simulink model "Fuzzy_System"  (R2024b)
settings: Solver=VariableStepAuto  StartTime=0.0  StopTime=10.0  RelTol=1e-3
values from neighbouring files (symbols this model uses):
  Age = 1    [main.m]
  Fixed_Expenses = 1    [main.m]
  Marital_Status = 1    [main.m]
  Num_Children = 1    [main.m]
  Real_Estate_Mortgage = 1    [main.m]
  Social = 1    [main.m]
libraries: fuzblock x3
settings Model: Creator=baley  LastModifiedBy=baley

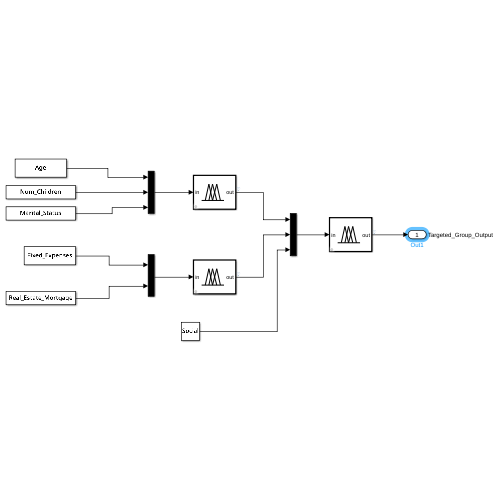
[thumbnail: Simulink's stored preview of the top-level diagram]
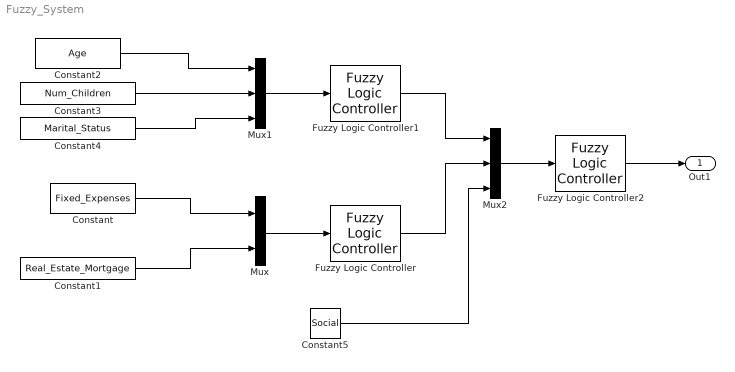
== system Fuzzy_System ==
  Constant : Constant  Value=Fixed_Expenses
  Constant1 : Constant  Value=Real_Estate_Mortgage
  Constant2 : Constant  Value=Age
  Constant3 : Constant  Value=Num_Children
  Constant4 : Constant  Value=Marital_Status
  Constant5 : Constant  Value=Social
  Fuzzy Logic Controller : fuzblock/Fuzzy Logic  Controller  FIS='financial_background.fis'  OutputSampleNumber=101  DataType=double  FuzzifiedInputs=off  RuleFiringStrengths=off  RuleOutputs=off  AggregatedOutputs=off  SimulateUsing=Interpreted execution  OutOfRangeInputValueMessage=warning  NoRuleFiredMessage=warning  EmptyOutputFuzzySetMessage=warning
  Fuzzy Logic Controller1 : fuzblock/Fuzzy Logic  Controller  FIS='personal_data.fis'  OutputSampleNumber=101  DataType=double  FuzzifiedInputs=off  RuleFiringStrengths=off  RuleOutputs=off  AggregatedOutputs=off  SimulateUsing=Interpreted execution  OutOfRangeInputValueMessage=warning  NoRuleFiredMessage=warning  EmptyOutputFuzzySetMessage=warning
  Fuzzy Logic Controller2 : fuzblock/Fuzzy Logic  Controller  FIS='targeted_group.fis'  OutputSampleNumber=101  DataType=double  FuzzifiedInputs=off  RuleFiringStrengths=off  RuleOutputs=off  AggregatedOutputs=off  SimulateUsing=Interpreted execution  OutOfRangeInputValueMessage=warning  NoRuleFiredMessage=warning  EmptyOutputFuzzySetMessage=warning
  Mux : Mux  Inputs=2
  Mux1 : Mux  Inputs=3
  Mux2 : Mux  Inputs=3
  Out1 : Outport  SignalName=Targeted_Group_Output
  wires:
  Mux/1 -> Fuzzy Logic Controller/1
  Constant/1 -> Mux/1
  Constant1/1 -> Mux/2
  Mux1/1 -> Fuzzy Logic Controller1/1
  Constant2/1 -> Mux1/1
  Constant3/1 -> Mux1/2
  Constant4/1 -> Mux1/3
  Fuzzy Logic Controller1/1 -> Mux2/1
  Fuzzy Logic Controller/1 -> Mux2/2
  Constant5/1 -> Mux2/3
  Mux2/1 -> Fuzzy Logic Controller2/1
  Fuzzy Logic Controller2/1 -> Out1/1
